simulink model "Lithium_ion_Battery_Model_with_and_without_Temperature_effect"  (R2021a)
settings: Solver=ode23tb  StartTime=0  StopTime=4000  MaxStep=0.1  RelTol=1e-4  EnableMultiTasking=on
undefined symbols (not defined in the file): Ion, Lithium
libraries: spsBatteryLib x2, spsControlledCurrentSourceLib x2, spsStairGeneratorLib x1, spspowerguiLib x1
settings Model: Creator=The MathWorks, Inc.  LastModifiedBy=siddi
settings SolverCC: AlgebraicLoopSolver=TrustRegion
settings DataIOCC: LimitDataPoints=on  SaveFormat=Array  ReturnWorkspaceOutputs=off
settings OptimizationCC: ExpressionDepthLimit=2147483647  InitFltsAndDblsToZero=on  LifeSpan=inf
settings DebuggingCC: UnderspecifiedInitializationDetection=Classic  MergeDetectMultiDrivingBlocksExec=none  SignalResolutionControl=TryResolveAllWithWarning  SolverPrmCheckMsg=warning  FcnCallInpInsideContextMsg=warning  AllowSymbolicDim=off  StateNameClashWarn=warning  SFUnexpectedBacktrackingDiag=warning  SFNoUnconditionalDefaultTransitionDiag=warning  SFExecutionAtInitializationDiag=none  SFMachineParentedDataDiag=warning  ArithmeticOperatorsInVariantConditions=warning
settings HardwareCC: ProdBitPerPointer=32  ProdBitPerSizeT=32  ProdBitPerPtrDiffT=32  ProdLargestAtomicFloat=None  ProdIntDivRoundTo=Undefined  ProdEndianess=Unspecified  ProdWordSize=32  ProdHWDeviceType=32-bit Generic
settings ModelReferenceCC: PropagateSignalLabelsOutOfModel=off
settings SFSimCC: SimUseLocalCustomCode=off  CustomCodeUndefinedFunction=UseInterfaceOnly
settings RTWCC: RTWUseLocalCustomCode=off
settings CodeAppCC: StateflowObjectComments=on
settings GRTTargetCC: TargetLangStandard=C89/C90 (ANSI)  CombineOutputUpdateFcns=off  GRTInterface=on
settings ConfigComp: CovMetricSettings=dw  CovSaveCumulativeToWorkspaceVar=on  CovSaveSingleToWorkspaceVar=on  CovExternalEMLEnable=off  CovSFcnEnable=off
settings SimscapeCC: SimscapeNormalizeSystem=off

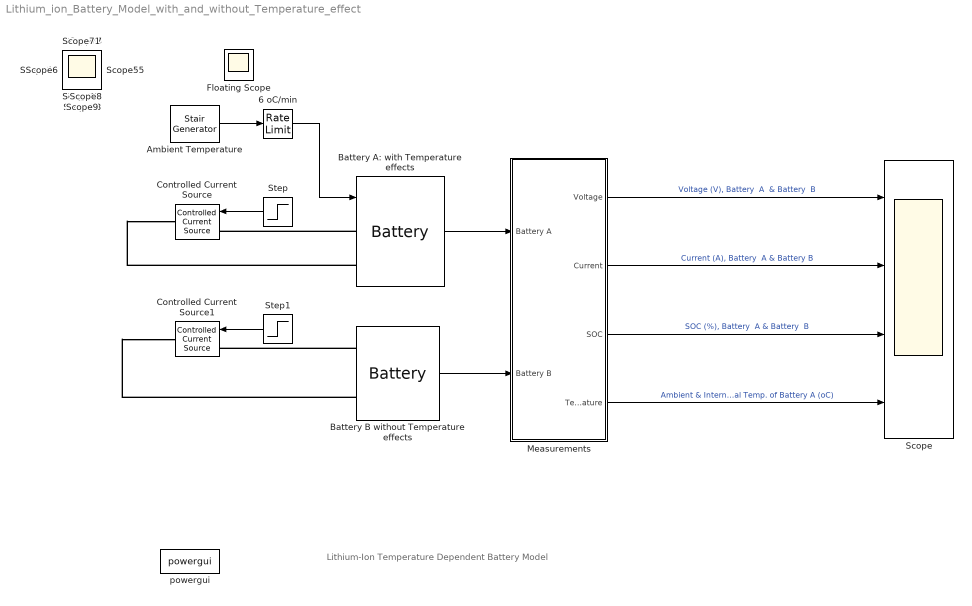
== system Lithium_ion_Battery_Model_with_and_without_Temperature_effect ==
  note: Lithium-Ion Temperature Dependent Battery Model
  6 oC/min : RateLimiter  RisingSlewLimit=0.5  FallingSlewLimit=-0.5  SampleTimeMode=inherited
  Ambient Temperature : spsStairGeneratorLib/Stair Generator  t="[0, 500, 1000 1500  2000 2500]"  e="[20, 20, -20  -20  0 0]"  Ts=0
  Battery A: with Temperature effects : spsBatteryLib/Battery  BatType=Lithium-Ion  ShowTempParam=on  ThermalPreset="7.4V  5.4Ah  (LiCoO2)"  ShowAgeParam=off  NomV=7  NomQ=5.4  SOC=100  Batt_Tr=30  PresetModel=off  MaxQ=5.6  MinV=5.25  FullV=8.3807  Dis_rate=1.1  R=0.0133  Normal_OP=5.2  expZone="[7.9           1]"  current=[6.5 13 32.5]  Units=Time  Tci=20  NomT=20  T2=-30  MaxQ2=4.8  FullV2=7.1  Normal_OP2=5.655  expZone2="[6.58           1]"  Rca=0.6  ti=2000  Dp=0  Neq0=0  Tsim=1e6  Ta1=25  Qeol=5.4*0.9  Reol=0.013333*1.2  Char_age=[2.3478, 3]  Dis_age=[2.3478, 10]  N1=1500  N2=10500  N3=1000  N4=1400  Ta2=45  N5=950
  Battery B without Temperature effects : spsBatteryLib/Battery  BatType=Lithium-Ion  ShowTempParam=off  ThermalPreset=no  ShowAgeParam=off  NomV=7  NomQ=5.4  SOC=100  Batt_Tr=30  PresetModel=off  MaxQ=5.6  MinV=5.25  FullV=8.3807  Dis_rate=1.1  R=0.0133  Normal_OP=5.2  expZone="[7.9    1]"  current=[6.5 13 32.5]  Units=Time  Tci=20  NomT=20  T2=-30  MaxQ2=4.8  FullV2=7.1  Normal_OP2=5.72  expZone2="[6.58  1]"  Rca=0.6  ti=1000  Dp=0  Neq0=0  Tsim=1e6  Ta1=25  Qeol=5.4*0.9  Reol=0.013333*1.2  Char_age=[2.3478, 3]  Dis_age=[2.3478, 10]  N1=1500  N2=10500  N3=1000  N4=1400  Ta2=45  N5=950
  Controlled Current Source : spsControlledCurrentSourceLib/Controlled Current Source  Initialize=on  Source_Type=AC  Amplitude=0  Phase=0  Frequency=0  Measurements=None
  Controlled Current Source1 : spsControlledCurrentSourceLib/Controlled Current Source  Initialize=on  Source_Type=AC  Amplitude=0  Phase=0  Frequency=0  Measurements=None
  Measurements : Subsystem
  "Scope " : Scope  NumInputPorts=4
  Step : Step  Time=2500  Before=2  After=-3  SampleTime=0
  Step1 : Step  Time=2500  Before=2  After=-3  SampleTime=0
  powergui : spspowerguiLib/powergui  SimulationMode=Continuous  SampleTime=0.001  frequency=60  Iterations=50  frequencyindice=0  Pbase=100e6  ErrMax=1e-4  UnitsV=kV  UnitsW=MW  buscounter=0  FunctionMessages=off  echomessages=off  EnableUseOfTLC=off  CurrentSourceSwitches=off  DisableSnubberDevices=off  DisableRonSwitches=off  DisableVfSwitches=off  DisplayEquations=off  AutomaticDiscreteSolvers=off  SolverType=Tustin  Interpol=off  ExternalGateDelay=off  methode=off  Ts=0  x0status=blocks  SPID=off  SwTol=0  HookPort=off  NonlinearTolerance=0  nMaxIteration=15  ContinueOnMaxIteration=off  RestoreLinks=warning  ResistiveCurrentMeasurement=off  Frange=[0:2:500]  Ylog=off  Xlog=on  ShowGrid=off  save=off  variable=ZData  structure=0  ZoomFFT=on  StartTime=0.0  cycles=1  DisplayStyle=1  fundamental=60  FreqAxis=off  MaxFrequency=1000  frequencyindicesteady=1  RmsSteady=1  display=off
  Floating Scope : Scope
  Scope{1..43} (43 alike) : Scope
  wires:
  Ambient Temperature/1 -> 6 oC/min/1
  6 oC/min/1 -> Battery A: with Temperature effects/1
  Step/1 -> Controlled Current Source/1
  Step1/1 -> Controlled Current Source1/1
  Battery A: with Temperature effects/1 -> Measurements/1(Battery A)
  Battery B without Temperature effects/1 -> Measurements/2(Battery B)
  Measurements/1(Voltage) -> "Scope "/1  "Voltage (V), Battery  A  & Battery  B"
  Measurements/2(Current) -> "Scope "/2  "Current (A), Battery  A & Battery B"
  Measurements/3(SOC) -> "Scope "/3  "SOC (%), Battery  A & Battery  B"
  Measurements/4(Temperature) -> "Scope "/4  "Ambient & Internal Temp. of Battery A (oC)"
  connections:
  Battery A: with Temperature effects/LConn2 -- Controlled Current Source/RConn1
  Battery A: with Temperature effects/LConn1 -- Controlled Current Source/LConn1
  Battery B without Temperature effects/LConn1 -- Controlled Current Source1/LConn1
  Battery B without Temperature effects/LConn2 -- Controlled Current Source1/RConn1

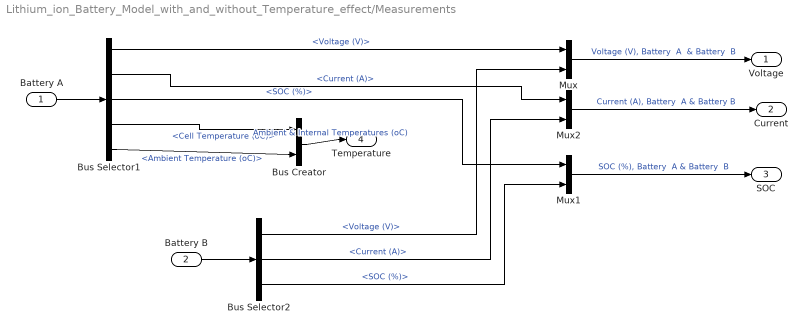
== system Lithium_ion_Battery_Model_with_and_without_Temperature_effect/Measurements ==
  Battery A : Inport
  Battery B : Inport  Port=2
  Bus Creator : BusCreator  Inputs=2
  Bus Selector1 : BusSelector  OutputSignals=Voltage (V),Current (A),SOC (%),Cell Temperature (oC),Ambient Temperature (oC)
  Bus Selector2 : BusSelector  OutputSignals=Voltage (V),Current (A),SOC (%)
  Mux : Mux  Inputs=2
  Mux1 : Mux  Inputs=2
  Mux2 : Mux  Inputs=2
  Voltage : Outport  VectorParamsAs1DForOutWhenUnconnected=off
  Current : Outport  Port=2  VectorParamsAs1DForOutWhenUnconnected=off
  SOC : Outport  Port=3  VectorParamsAs1DForOutWhenUnconnected=off
  Temperature : Outport  Port=4  VectorParamsAs1DForOutWhenUnconnected=off
  wires:
  Bus Selector1/4 -> Bus Creator/1  "<Cell Temperature (oC)>"
  Bus Selector1/5 -> Bus Creator/2  "<Ambient Temperature (oC)>"
  Bus Creator/1 -> Temperature/1  "Ambient & Internal Temperatures (oC)"
  Bus Selector1/3 -> Mux1/1  "<SOC (%)>"
  Battery B/1 -> Bus Selector2/1
  Bus Selector2/3 -> Mux1/2  "<SOC (%)>"
  Mux1/1 -> SOC/1  "SOC (%), Battery  A & Battery  B"
  Mux/1 -> Voltage/1  "Voltage (V), Battery  A  & Battery  B"
  Bus Selector2/1 -> Mux/2  "<Voltage (V)>"
  Bus Selector1/1 -> Mux/1  "<Voltage (V)>"
  Bus Selector1/2 -> Mux2/1  "<Current (A)>"
  Bus Selector2/2 -> Mux2/2  "<Current (A)>"
  Mux2/1 -> Current/1  "Current (A), Battery  A & Battery B"
  Battery A/1 -> Bus Selector1/1
